simulink model "test_scheme"  (R2021b)
settings: Solver=VariableStepAuto  StartTime=0.0  StopTime=30  RelTol=1e-3
values from neighbouring files (symbols this model uses):
  H = 0    [design_state_controller_link_side.m]
  K = [-k1 k1 0 0 ... (first row only)    [DOF2_sea_model.m]    (also in design_state_controller_link_side.m = Khat(:,1:n))
  Ts = 1e-3    (= 0.001)    [design_state_controller_link_side.m]    (also in freq_resp_collabot.m; freq_resp_collabot_jnt2.m; freq_resp_collabot_jnt2_siso.m; joint3_collabot_ident.m)
libraries: simulink x1, cstblocks x1
settings Model: Creator=jacobi  LastModifiedBy=manue

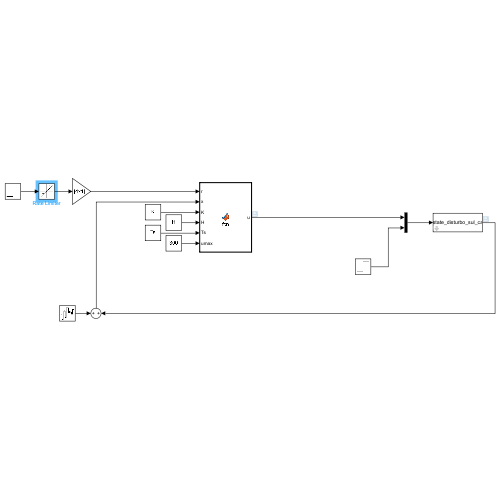
[thumbnail: Simulink's stored preview of the top-level diagram]
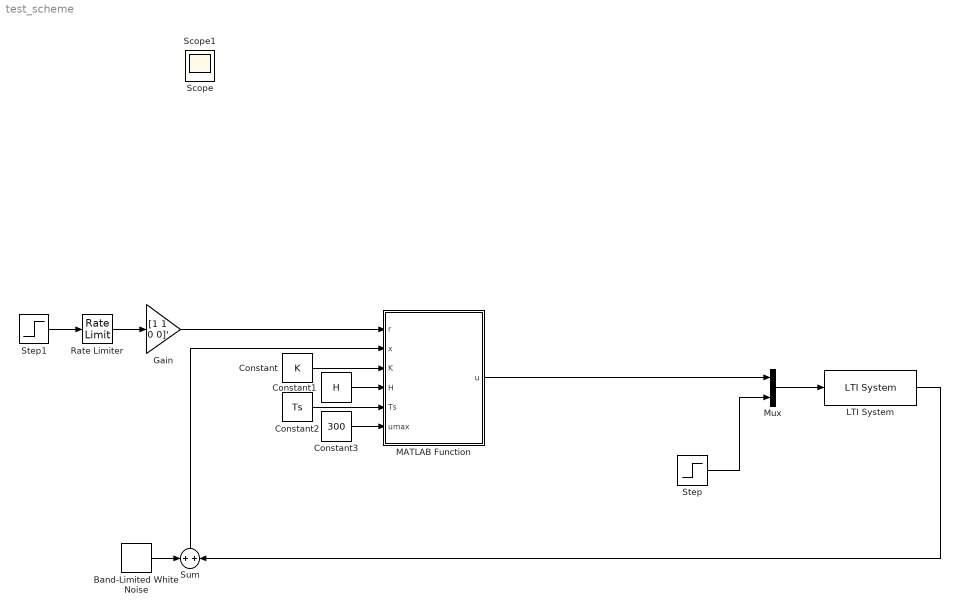
== system test_scheme ==
  Band-Limited White Noise : simulink/Sources/Band-Limited White Noise  Cov=[1e-6 1e-6 1e-3 1e-3]*1e-3  Ts=Ts  seed=[23341]
  Constant : Constant  Value=K
  Constant1 : Constant  Value=H
  Constant2 : Constant  Value=Ts
  Constant3 : Constant  Value=300
  Gain : Gain  Gain=[1 1 0 0]'
  LTI System : cstblocks/LTI System  sys=full_state_disturbo_sul_carico  IC=[]
  MATLAB Function : MATLAB Function  TreatAsAtomicUnit=on  SystemSampleTime=Ts
  Mux : Mux  Inputs=2
  Rate Limiter : RateLimiter  RisingSlewLimit=0.2  FallingSlewLimit=-0.2  SampleTimeMode=inherited
  Step : Step  Time=10  After=50  SampleTime=0
  Step1 : Step  SampleTime=0
  Sum : Sum
  Scope : Scope
  Scope1 : Scope
  wires:
  Mux/1 -> LTI System/1
  Step/1 -> Mux/2
  LTI System/1 -> Sum/2
  Step1/1 -> Rate Limiter/1
  MATLAB Function/1(u) -> Mux/1
  Constant/1 -> MATLAB Function/3(K)
  Constant1/1 -> MATLAB Function/4(H)
  Constant2/1 -> MATLAB Function/5(Ts)
  Constant3/1 -> MATLAB Function/6(umax)
  Band-Limited White Noise/1 -> Sum/1
  Sum/1 -> MATLAB Function/2(x)
  Gain/1 -> MATLAB Function/1(r)
  Rate Limiter/1 -> Gain/1

== matlab function test_scheme/MATLAB Function ==
  data: r input; u output; x input; K input; H input; Ts input; umax input
function u = fcn(r,x,K,H,Ts,umax)
persistent xi
if isempty(xi)
    xi=0;
end

u=K'*(r-x)+xi;
e=r(2)-x(2);
if (u>umax)
    u=umax;
    if (e<0)
        xi=xi+H*e*Ts;
    end
elseif (u<-umax)
    u=-umax;
    if (e>0)
        xi=xi+H*e*Ts;
    end
else
    xi=xi+H*e*Ts;
end
